simulink model "dus4_2"  (R2014a)
settings: Solver=FixedStepDiscrete  StartTime=0.0  StopTime=10.0  FixedStep=0.1  RelTol=1e-3
settings Model: Creator=yoshi12  LastModifiedBy=yoshi12

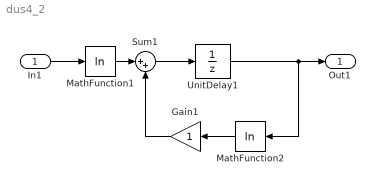
== system dus4_2 ==
  In1 : Inport
  Gain1 : Gain
  MathFunction1 : Math  Operator=log  SaturateOnIntegerOverflow=on
  MathFunction2 : Math  Operator=log  SaturateOnIntegerOverflow=on
  Sum1 : Sum  Inputs=|++
  UnitDelay1 : UnitDelay  SampleTime=-1
  Out1 : Outport
  wires:
  MathFunction1/1 -> Sum1/1
  UnitDelay1/1 -> Out1/1, MathFunction2/1
  Sum1/1 -> UnitDelay1/1
  In1/1 -> MathFunction1/1
  Gain1/1 -> Sum1/2
  MathFunction2/1 -> Gain1/1
